simulink model "speed_sensor_filter"  (R2024b)
settings: Solver=VariableStepAuto  StartTime=0.0  StopTime=10.0  RelTol=1e-3
undefined symbols (not defined in the file): Fw, incenc
settings Model: Creator=matth  LastModifiedBy=matth

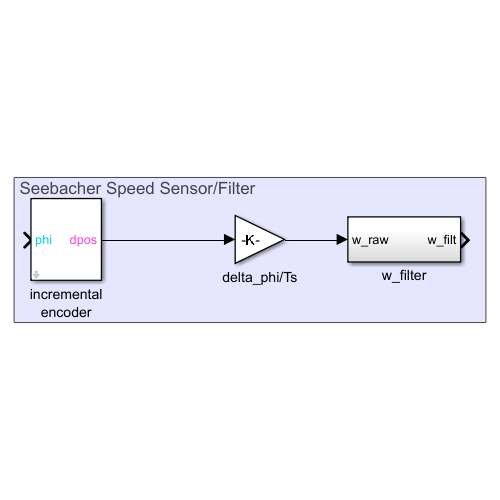
[thumbnail: Simulink's stored preview of the top-level diagram]
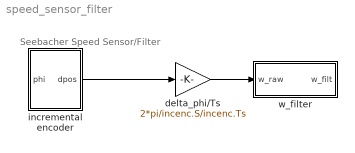
== system speed_sensor_filter ==
  note: Seebacher Speed Sensor/Filter
  delta_phi/Ts : Gain  Gain=2*pi/incenc.S/incenc.Ts  SaturateOnIntegerOverflow=on  OutDataTypeStr=Inherit: Same as input  ParamDataTypeStr=Inherit: Same as input
  incremental encoder : Subsystem  mask{incenc=incenc}
      mask prompts: incenc "Parameterstruct"
  w_filter : Subsystem
  wires:
  incremental encoder/1(dpos) -> delta_phi/Ts/1
  delta_phi/Ts/1 -> w_filter/1(w_raw)

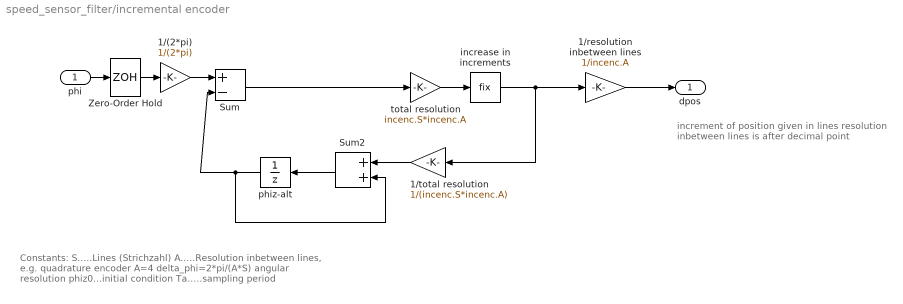
== system speed_sensor_filter/incremental encoder ==
  note: increment of position given in lines
      | resolution inbetween lines is after decimal point
  note: Constants:
      | S.....Lines (Strichzahl)
      | A.....Resolution inbetween lines, e.g. quadrature encoder A=4
      |        delta_phi=2*pi/(A*S) angular resolution
      | phiz0...initial condition
      | Ta.....sampling period
  phi : Inport
  1/(2*pi) : Gain  Gain=1/(2*pi)  OutDataTypeStr=Inherit: Same as input  ParamDataTypeStr=Inherit: Same as input
  1/resolution inbetween lines : Gain  Gain=1/incenc.A  OutDataTypeStr=Inherit: Same as input  ParamDataTypeStr=Inherit: Same as input
  1/total resolution : Gain  Gain=1/(incenc.S*incenc.A)  OutDataTypeStr=Inherit: Same as input  ParamDataTypeStr=Inherit: Same as input
  Sum : Sum  Inputs=+-  InputSameDT=on  OutDataTypeStr=Inherit: Same as first input
  Sum2 : Sum  InputSameDT=on  OutDataTypeStr=Inherit: Same as first input
  Zero-Order Hold : ZeroOrderHold  SampleTime=incenc.Ts
  increase in increments : Rounding  Operator=fix
  phiz-alt : UnitDelay  InitialCondition=incenc.phiz0  SampleTime=incenc.Ts  HasFrameUpgradeWarning=on
  total resolution : Gain  Gain=incenc.S*incenc.A  OutDataTypeStr=Inherit: Same as input  ParamDataTypeStr=Inherit: Same as input
  dpos : Outport  VectorParamsAs1DForOutWhenUnconnected=off
  wires:
  Sum2/1 -> phiz-alt/1
  1/total resolution/1 -> Sum2/1
  1/(2*pi)/1 -> Sum/1
  increase in increments/1 -> 1/resolution inbetween lines/1, 1/total resolution/1
  phi/1 -> Zero-Order Hold/1
  phiz-alt/1 -> Sum2/2, Sum/2
  total resolution/1 -> increase in increments/1
  Sum/1 -> total resolution/1
  Zero-Order Hold/1 -> 1/(2*pi)/1
  1/resolution inbetween lines/1 -> dpos/1

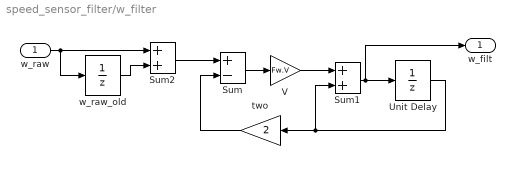
== system speed_sensor_filter/w_filter ==
  w_raw : Inport
  Sum : Sum  Inputs=+-  SaturateOnIntegerOverflow=on
  Sum1 : Sum  SaturateOnIntegerOverflow=on
  Sum2 : Sum  SaturateOnIntegerOverflow=on
  Unit Delay : UnitDelay  InitialCondition=Fw.w0  SampleTime=Fw.Ts  HasFrameUpgradeWarning=on
  V : Gain  Gain=Fw.V  SaturateOnIntegerOverflow=on  OutDataTypeStr=Inherit: Same as input  ParamDataTypeStr=Inherit: Same as input
  two : Gain  Gain=2  SaturateOnIntegerOverflow=on  OutDataTypeStr=Inherit: Same as input  ParamDataTypeStr=Inherit: Same as input
  w_raw_old : UnitDelay  InitialCondition=Fw.w0  SampleTime=Fw.Ts  HasFrameUpgradeWarning=on
  w_filt : Outport  VectorParamsAs1DForOutWhenUnconnected=off
  wires:
  Sum1/1 -> Unit Delay/1, w_filt/1
  Sum/1 -> V/1
  Sum2/1 -> Sum/1
  V/1 -> Sum1/1
  two/1 -> Sum/2
  Unit Delay/1 -> two/1, Sum1/2
  w_raw_old/1 -> Sum2/2
  w_raw/1 -> w_raw_old/1, Sum2/1
